simulink subsystem "medidor_velocidadcondist"  (R2023b)
settings: Solver=VariableStepAuto  StartTime=0.0  StopTime=10.0  RelTol=1e-3
libraries: arduinosensorlib x2, simulink x1
settings Model: Creator=juana  LastModifiedBy=juana

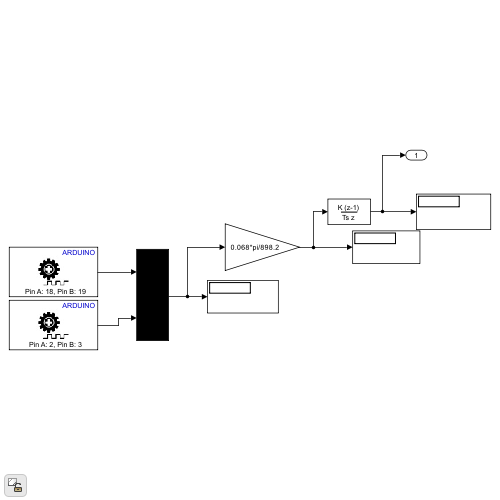
[thumbnail: Simulink's stored preview of the top-level diagram]
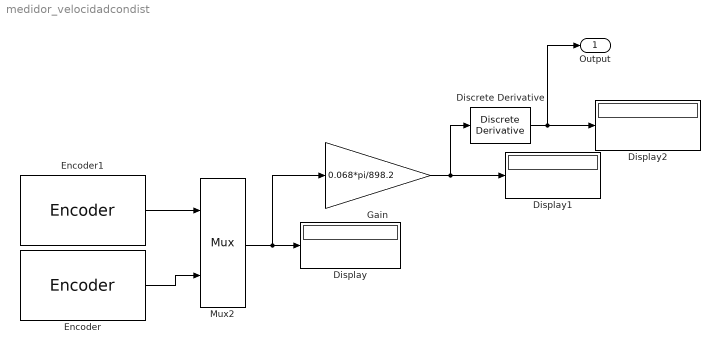
== system medidor_velocidadcondist ==
  Discrete Derivative : simulink/Discrete/Discrete Derivative  gainval=1.0  ICPrevScaledInput=0.0  OutMin=[]  OutMax=[]  OutDataType=fixdt(1, 16)  OutScaling=2^-10  DoSatur=off
  Display : Display
  Display1 : Display
  Display2 : Display
  Encoder : arduinosensorlib/Encoder  InputA=2  InputB=3  Mode=No reset  SampleTime=-1
  Encoder1 : arduinosensorlib/Encoder  InputA=18  InputB=19  Mode=No reset  SampleTime=-1
  Gain : Gain  Gain=0.068*pi/898.2
  Mux2 : Mux  Inputs=2
  Output : Outport
  wires:
  Discrete Derivative/1 -> Display2/1, Output/1
  Encoder1/1 -> Mux2/1
  Mux2/1 -> Display/1, Gain/1
  Encoder/1 -> Mux2/2
  Gain/1 -> Display1/1, Discrete Derivative/1
